simulink model "bayes_filter"  (R2025b)
settings: Solver=FixedStepAuto  StartTime=0.0  StopTime=15  FixedStep=0.01  RelTol=1e-3
values from neighbouring files (symbols this model uses):
  A = [1 0.01;-0.25 0.85]    [StateSpaceMatrices.m]
  B = [0;0.05]    [StateSpaceMatrices.m]
  C = [1 0;0 1]    [StateSpaceMatrices.m]
  D = [0;0]    [StateSpaceMatrices.m]
undefined symbols (not defined in the file or in its folder): Discrete, Time
libraries: simulink x2, ctrlSharedLib x1
settings Model: Creator=hussein  LastModifiedBy=hussein

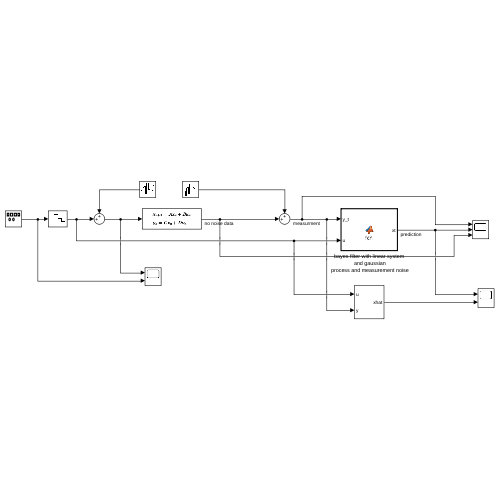
[thumbnail: Simulink's stored preview of the top-level diagram]
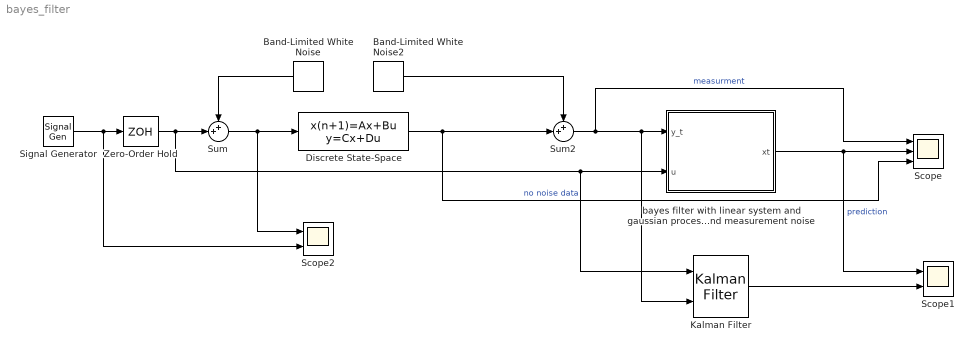
== system bayes_filter ==
  Band-Limited White Noise : simulink/Sources/Band-Limited White Noise  Cov=0.00008  Ts=0.01  seed=[23341]
  Band-Limited White Noise2 : simulink/Sources/Band-Limited White Noise  Cov=0.0005  Ts=0.01  seed=[23341]
  Discrete State-Space : DiscreteStateSpace  A=A  B=B  C=C  D=D  SampleTime=-1
  Kalman Filter : ctrlSharedLib/Kalman Filter  TimeDomain=Discrete-Time  UseCurrentEstimator=on  ModelSource=Individual A, B, C, D matrices  ModelSourceVariable=ss(0.95,1,1,0,1)  A=A  B=B  C=C  D=D  NumberOfStates=1  NumberOfInputs=1  NumberOfOutputs=1  InitialEstimateSource=Dialog  X0=0  P0=10  UseK=off  UseGH=off  NumberOfProcessNoiseInputs=1  G=1  TimeInvariantG=on  H=0  TimeInvariantH=on  Q=|  TimeInvariantQ=on  R=[5 0;0 5]  TimeInvariantR=on  N=0  TimeInvariantN=on  AddInputPort=on  AddEnablePort=off  OutputEstimatedY=off  OutputP=off  Ts=-1
      | [0.0003 0;
      |    0 0.0003]
  Scope : Scope  NumInputPorts=3
      settings: ActiveDisplayYMinimum=-1.2172616775034109  ActiveDisplayYMaximum=1.2097576273363002
  Scope1 : Scope  NumInputPorts=2
      settings: ActiveDisplayYMinimum=-0.26322769799515411  ActiveDisplayYMaximum=0.44790813131940238
  Scope2 : Scope  NumInputPorts=2
      settings: ActiveDisplayYMinimum=-1.5096055747769204  ActiveDisplayYMaximum=1.7514023036159916  DataLoggingVariableName=ScopeData2
  Signal Generator : SignalGenerator  WaveForm=sawtooth  Frequency=pi  Units=rad/sec
  Sum : Sum  Inputs=++|
  Sum2 : Sum  Inputs=++|
  Zero-Order Hold : ZeroOrderHold  SampleTime=0.01
  bayes filter with linear system and gaussian process and measurement noise : MATLAB Function  TreatAsAtomicUnit=on
  wires:
  Band-Limited White Noise2/1 -> Sum2/1
  Sum/1 -> Scope2/1, Discrete State-Space/1
  bayes filter with linear system and gaussian process and measurement noise/1(xt) -> Scope1/1, Scope/2  "prediction"
  Band-Limited White Noise/1 -> Sum/1
  Sum2/1 -> Kalman Filter/2, bayes filter with linear system and gaussian process and measurement noise/1(y_t), Scope/1  "measurment"
  Zero-Order Hold/1 -> Kalman Filter/1, bayes filter with linear system and gaussian process and measurement noise/2(u), Sum/2
  Discrete State-Space/1 -> Sum2/2, Scope/3  "no noise data"
  Signal Generator/1 -> Scope2/2, Zero-Order Hold/1
  Kalman Filter/1 -> Scope1/2

== matlab function bayes_filter/bayes filter with linear system and gaussian process and measurement noise ==
  data: y_t input; u input; xt output
function xt = fcn(y_t, u)

persistent bel_previous

A=[1 0.01;-0.25 0.85];
B=[0;0.05];
C=[1 0;0 1];
D=[0;0];
Q=[0.0003 0;
   0 0.0003];
R=[5 0;
   0 5];

if isempty(bel_previous)
    bel_previous.mean = [0;0];
    bel_previous.cov  = [0 0; 0 0];
end

% -------- Prediction --------
bel_bar.mean = A*bel_previous.mean + B*u;
bel_bar.cov  = A*bel_previous.cov*A' + Q;

% -------- Correction --------
bel.mean = zeros(2,1);     
bel.cov  = zeros(2,2);
bel.cov  = inv(inv(bel_bar.cov) + C'*inv(R)*C);
bel.mean = bel.cov * (C'*inv(R)*y_t + inv(bel_bar.cov)*bel_bar.mean);

% -------- Normalizing --------
eta_rec.mean = zeros(2,1);     
eta_rec.cov  = zeros(2,2);
bel_norm.mean = zeros(2,1);     
bel_norm.cov  = zeros(2,2);

eta_rec.mean=C*bel_bar.mean;
eta_rec.cov=C*bel_bar.cov*C'+R;

bel_norm.cov=inv(inv(bel.cov)-inv(eta_rec.cov));
bel_norm.mean=bel_norm.cov*(inv(bel.cov)*bel.mean-inv(eta_rec.cov)*eta_rec.mean);


% -------- Update Persistent --------
bel_previous=bel_norm;


xt = bel_norm.mean;
